simulink model "pid_ziegler"  (R2023a)
settings: Solver=VariableStepAuto  StartTime=0.0  StopTime=10.0  RelTol=1e-3
settings Model: Creator=omega  LastModifiedBy=omega

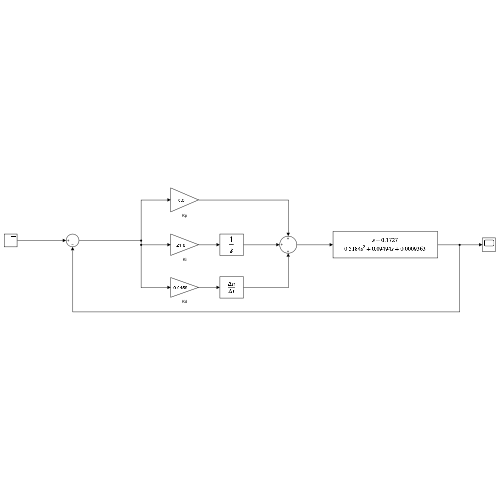
[thumbnail: Simulink's stored preview of the top-level diagram]
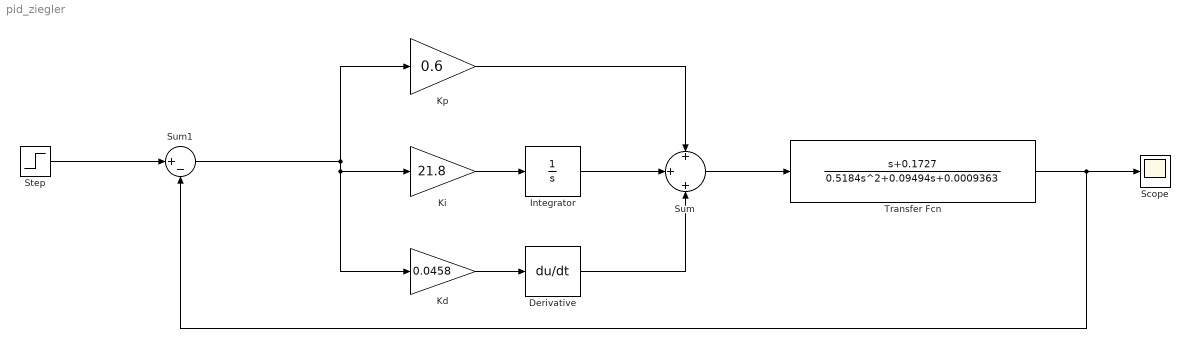
== system pid_ziegler ==
  Derivative : Derivative
  Integrator : Integrator
  Kd : Gain  Gain=0.0458
  Ki : Gain  Gain=21.8
  Kp : Gain  Gain=0.6
  Scope : Scope
  Step : Step  SampleTime=0
  Sum : Sum  Inputs=+||+||+
  Sum1 : Sum  Inputs=|+-
  Transfer Fcn : TransferFcn  Numerator=[1 0.1727]  Denominator=[0.5184 0.09494 0.0009363]
  wires:
  Kp/1 -> Sum/1
  Integrator/1 -> Sum/2
  Derivative/1 -> Sum/3
  Kd/1 -> Derivative/1
  Ki/1 -> Integrator/1
  Sum/1 -> Transfer Fcn/1
  Step/1 -> Sum1/1
  Sum1/1 -> Kd/1, Ki/1, Kp/1
  Transfer Fcn/1 -> Scope/1, Sum1/2
